simulink model "LibraryExample"  (R2017a)
settings: Solver=VariableStepAuto  StartTime=0.0  StopTime=10.0  RelTol=1e-3
libraries: TestLibrary x2
settings Model: Creator=ptracton  LastModifiedBy=ptracton

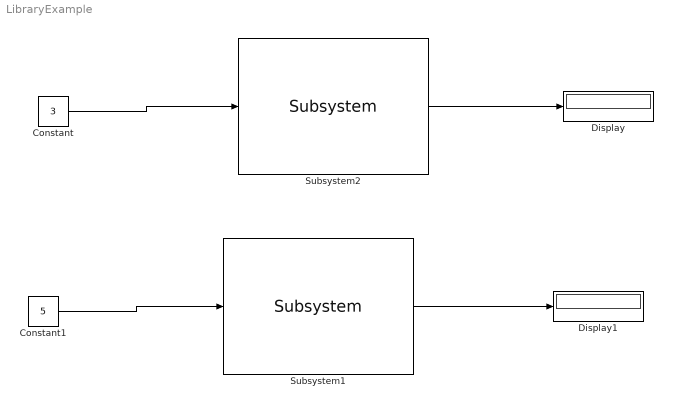
== system LibraryExample ==
  Constant : Constant  Value=3
  Constant1 : Constant  Value=5
  Display : Display
  Display1 : Display
  Subsystem1 : TestLibrary/Subsystem
  Subsystem2 : TestLibrary/Subsystem
  wires:
  Constant/1 -> Subsystem2/1
  Subsystem2/1 -> Display/1
  Constant1/1 -> Subsystem1/1
  Subsystem1/1 -> Display1/1
